simulink model "bTestModelOLD"  (R2015a)
settings: Solver=ode45  StartTime=0.0  StopTime=12  RelTol=1e-6
values from neighbouring files (symbols this model uses):
  B_f = 7.4e-3    (= 0.0074)    [bTestComparison.m]
  g = 9.82    [bTestComparison.m]
  J_f = 5.6e-3    (= 0.0056)    [bTestComparison.m]
  J_w = 0.601e-3    (= 0.000601)    [bTestComparison.m]
  l_f = 0.08498    [bTestComparison.m]
  l_w = 0.093    [bTestComparison.m]
  m_f = 0.77-m_w    (= 0.548)    [bTestComparison.m]
  m_w = 0.222    [bTestComparison.m]
settings Model: CovSFcnEnable=off  Creator=USUARIO  LastModifiedBy=USUARIO
settings DataIOCC: LimitDataPoints=off
settings DebuggingCC: SolverPrmCheckMsg=warning

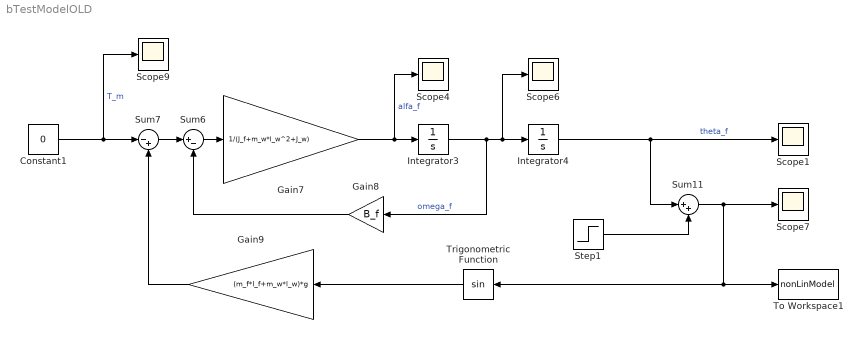
== system bTestModelOLD ==
  Constant1 : Constant  Value=0
  Gain7 : Gain  Gain=1/(J_f+m_w*l_w^2+J_w)
  Gain8 : Gain  Gain=B_f
  Gain9 : Gain  Gain=(m_f*l_f+m_w*l_w)*g
  Integrator3 : Integrator
  Integrator4 : Integrator
  Scope{1,4,6..7,9} (5 alike) : Scope
      Scope1 settings: TimeRange=2  LimitDataPoints=on  MaxDataPoints=5000  SaveName=StepResponseData  YMin=0  YMax=14000  SampleTime=-1
      Scope4 settings: TimeRange=auto  LimitDataPoints=on  MaxDataPoints=5000  SaveToWorkspace=off  SaveName=ScopeData2  YMin=-10  YMax=10  SampleTime=-1
      Scope6 settings: TimeRange=auto  LimitDataPoints=on  MaxDataPoints=5000  SaveToWorkspace=off  SaveName=ScopeData4  YMin=-10  YMax=10  SampleTime=-1
      Scope7 settings: TimeRange=2  LimitDataPoints=on  MaxDataPoints=5000  SaveName=StepResponseData1  YMin=0  YMax=14000  SampleTime=-1
      Scope9 settings: TimeRange=auto  LimitDataPoints=on  MaxDataPoints=5000  SaveToWorkspace=off  SaveName=ScopeData7  YMin=-10  YMax=10  SampleTime=-1
  Step1 : Step  Time=0  After=pi/2+pi/4  SampleTime=0
  Sum11 : Sum  Inputs=|++
  Sum6 : Sum  Inputs=|+-
  Sum7 : Sum  Inputs=|-+
  To Workspace1 : ToWorkspace  VariableName=nonLinModel  SaveFormat=Timeseries  SampleTime=-1
  Trigonometric Function : Trigonometry
  wires:
  Gain7/1 -> Scope4/1, Integrator3/1  "alfa_f"
  Integrator3/1 -> Gain8/1, Scope6/1, Integrator4/1  "omega_f"
  Sum6/1 -> Gain7/1
  Sum7/1 -> Sum6/1
  Gain8/1 -> Sum6/2
  Gain9/1 -> Sum7/2
  Constant1/1 -> Sum7/1, Scope9/1  "T_m"
  Integrator4/1 -> Scope1/1, Sum11/1  "theta_f"
  Step1/1 -> Sum11/2
  Sum11/1 -> Scope7/1, Trigonometric Function/1, To Workspace1/1
  Trigonometric Function/1 -> Gain9/1
